simulink model "Refined_Model_42_VectoTnT"  (R2020b)
settings: Solver=FixedStepAuto  StartTime=0.0  StopTime=2500  FixedStep=dt  RelTol=1e-3
values from neighbouring files (symbols this model uses):
  ALInpSpeed = AxlLoss (1,:)    [GPS_val.m]    (also in ICEBEV_Script.m; ICEBEV_Script_VECTO.m; ICE_Script.m; ICE_Script_SSVal.m)
  ALInpTor = AxlLoss(:,1)    [GPS_val.m]    (also in ICEBEV_Script.m; ICEBEV_Script_VECTO.m; ICE_Script.m; ICE_Script_SSVal.m)
  ALTableVal = AxlLoss(2:end,2:end)    [GPS_val.m]    (also in ICEBEV_Script.m; ICEBEV_Script_VECTO.m; ICE_Script.m; ICE_Script_SSVal.m)
  CovDist = RoadProfile(:,4)    [ICE_Val.m]
  Cx = VehicleDefine(7,3)    [BEV_Basictest.m]    (also in GPS_val.m; ICEBEV_Script.m; ICEBEV_Script_VECTO.m; ICE_Script.m)
  Dist = 1:length(MaxSpeedProfile)    [GPS_val.m]    (also in ICE_Script.m; ICE_Val.m = [1:CovDist(end)])
  DynRolRad = VehicleDefine(5,3)    [BEV_Basictest.m]    (also in GPS_val.m; ICEBEV_Script.m; ICEBEV_Script_VECTO.m; ICE_Script.m)
  EngineRpm = round(IntpTorCur(:,1))    [GPS_val.m]    (also in ICEBEV_Script.m; ICEBEV_Script_VECTO.m; ICE_Script.m; ICE_Script_SSVal.m)
  EngineRpmRaw = TorCurRaw(:,1)    [GPS_val.m]    (also in ICEBEV_Script.m; ICEBEV_Script_VECTO.m; ICE_Script.m; ICE_Script_SSVal.m)
  etaClutch = VehicleDefine(23,3)    [GPS_val.m]    (also in ICEBEV_Script.m; ICEBEV_Script_VECTO.m; ICE_Script.m; ICE_Script_SSVal.m)
  FCTableVal = FCMap(2:end,2:end)    [GPS_val.m]    (also in ICEBEV_Script.m; ICEBEV_Script_VECTO.m; ICE_Script.m; ICE_Script_SSVal.m)
  FDR = VehicleDefine(20,3)    [BEV_Basictest.m]    (also in GPS_val.m = VehicleDefine(22,3); ICEBEV_Script.m = VehicleDefine(22,3); ICEBEV_Script_VECTO.m = VehicleDefine(22,3); ICE_Script.m = VehicleDefine(22,3))
  Fr = VehicleDefine(13,3)    [BEV_Basictest.m]    (also in GPS_val.m; ICEBEV_Script.m; ICEBEV_Script_VECTO.m; ICE_Script.m)
  g = VehicleDefine(14,3)    [BEV_Basictest.m]    (also in GPS_val.m; ICEBEV_Script.m; ICEBEV_Script_VECTO.m; ICE_Script.m)
  GNo = GBXDefine(:,1)    [GPS_val.m]    (also in ICEBEV_Script.m; ICEBEV_Script_VECTO.m; ICE_Script.m; ICE_Script_SSVal.m)
  GRa = GBXDefine(:,2)    [GPS_val.m]    (also in ICEBEV_Script.m; ICEBEV_Script_VECTO.m; ICE_Script.m; ICE_Script_SSVal.m)
  InitVel = VehicleDefine(21,3)    [BEV_Basictest.m]    (also in GPS_val.m = VehicleDefine(24,3); ICEBEV_Script.m = VehicleDefine(24,3); ICEBEV_Script_VECTO.m = VehicleDefine(24,3); ICE_Script.m = VehicleDefine(24,3))
  IntpSlope = round(IntpSlope,1)    [GPS_val.m]    (also in ICE_Script.m; ICE_Val.m = A)
  Je = VehicleDefine(25,3)    [GPS_val.m]    (also in ICEBEV_Script.m; ICEBEV_Script_VECTO.m; ICE_Script.m; ICE_Script_SSVal.m)
  Jk = VehicleDefine(15,3)    [BEV_Basictest.m]    (also in GPS_val.m; ICEBEV_Script.m; ICEBEV_Script_VECTO.m; ICE_Script.m)
  Jm = VehicleDefine(16,3)    [GPS_val.m]    (also in ICEBEV_Script.m; ICEBEV_Script_VECTO.m; ICE_Script.m; ICE_Script_SSVal.m)
  MaxAcc = 1    [BEV_Basictest.m]    (also in GPS_val.m; ICEBEV_Script.m; ICEBEV_Script_VECTO.m; ICE_Script.m)
  MaxDec = 1    [BEV_Basictest.m]    (also in GPS_val.m; ICEBEV_Script.m; ICEBEV_Script_VECTO.m; ICE_Script.m)
  MaxSpeedProfile = FMSP    [GPS_val.m]    (also in ICE_Script.m; ICE_Val.m = repelem(SegSPLatinmps,SegLeninm))
  MaxTorValThrot = max(ThrotTableVal,[],2)    [GPS_val.m]    (also in ICEBEV_Script.m; ICEBEV_Script_VECTO.m; ICE_Script.m; ICE_Script_SSVal.m)
  Me = VehicleDefine(10,3)    [BEV_Basictest.m]    (also in GPS_val.m; ICEBEV_Script.m; ICEBEV_Script_VECTO.m; ICE_Script.m)
  MotoringTor = IntpTorCur(:,3)    [GPS_val.m]    (also in ICEBEV_Script.m; ICEBEV_Script_VECTO.m; ICE_Script.m; ICE_Script_SSVal.m)
  Mt = VehicleDefine(12,3)    [BEV_Basictest.m]    (also in GPS_val.m; ICEBEV_Script.m; ICEBEV_Script_VECTO.m; ICE_Script.m)
  Mtot = Mv+Me+Mt    [BEV_Basictest.m]    (also in GPS_val.m; ICEBEV_Script.m; ICEBEV_Script_VECTO.m; ICE_Script.m)
  Mv = VehicleDefine(9,3)    [BEV_Basictest.m]    (also in GPS_val.m; ICEBEV_Script.m; ICEBEV_Script_VECTO.m; ICE_Script.m)
  NoSteps = round(Dist(end))    [GPS_val.m]    (also in ICE_Script.m; ICE_Val.m = 3002)
  NoWhlFA = VehicleDefine(2,3)    [BEV_Basictest.m]    (also in GPS_val.m; ICE_Script.m; ICE_Val.m; ICE_Val_new.m)
  NoWhlRA = VehicleDefine(4,3)    [BEV_Basictest.m]    (also in GPS_val.m; ICE_Script.m; ICE_Val.m; ICE_Val_new.m)
  rho = VehicleDefine(6,3)    [BEV_Basictest.m]    (also in GPS_val.m; ICEBEV_Script.m; ICEBEV_Script_VECTO.m; ICE_Script.m)
  RpmBrkPnt = ThrottleMap(1,:)    [GPS_val.m]    (also in ICEBEV_Script.m; ICEBEV_Script_VECTO.m; ICE_Script.m; ICE_Script_SSVal.m)
  s = divisors(length(MaxSpeedProfile))    [GPS_val.m]    (also in ICEBEV_Script.m = round(FLoadTor); ICEBEV_Script_VECTO.m = round(FLoadTor); ICE_Script.m = round(FLoadTor); ICE_Script_SSVal.m = round(FLoadTor))
  SegNo = RoadProfile(:,1)    [ICE_Val.m]
  SegSPLatinmps = (sqrt(aMaxLat*g*CurRadinm))    [GPS_val.m]    (also in ICE_Script.m; ICE_Val.m)
  Sx = VehicleDefine(8,3)    [BEV_Basictest.m]    (also in GPS_val.m; ICEBEV_Script.m; ICEBEV_Script_VECTO.m; ICE_Script.m)
  ThrotPos = ThrotPos'    [GPS_val.m]    (also in ICEBEV_Script.m; ICEBEV_Script_VECTO.m; ICE_Script.m; ICE_Script_SSVal.m)
  ThrotTableVal = ThrottleMap(2:end,2:end)    [GPS_val.m]    (also in ICEBEV_Script.m; ICEBEV_Script_VECTO.m; ICE_Script.m; ICE_Script_SSVal.m)
undefined symbols (not defined in the file or in its folder): G1Inprpm, GearNo, GInprpm, GInpTor, GTorLoss, MaxSpinG, MaxWhlTorinG, Stoptimes
libraries: simulink x4, autolibshared x1
settings Model: Creator=Kshitij  LastModifiedBy=Kshitij
settings DebuggingCC: AlgebraicLoopMsg=none

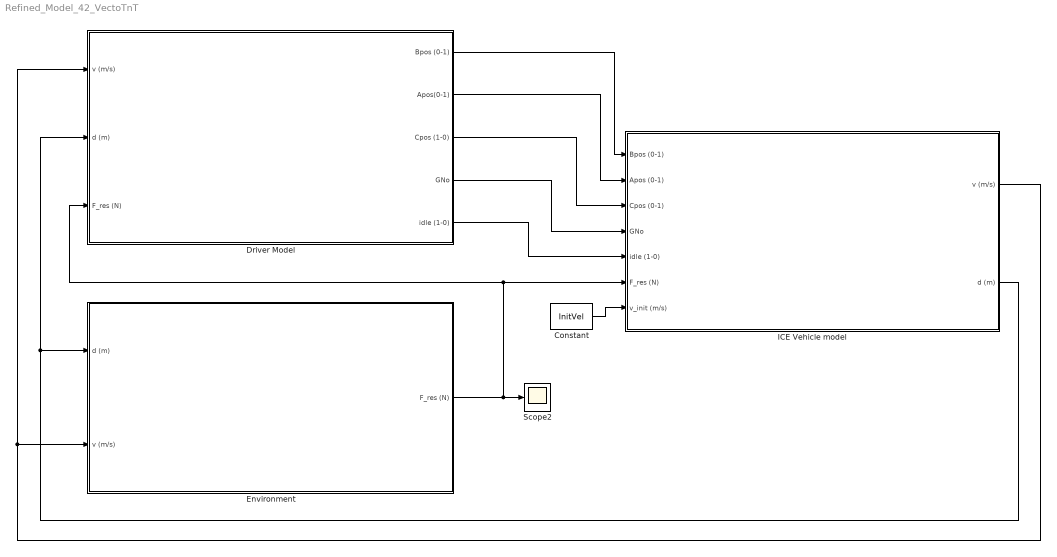
== system Refined_Model_42_VectoTnT ==
  Constant : Constant  Value=InitVel
  Driver Model : Subsystem
  Environment : Subsystem
  ICE Vehicle model : Subsystem
  Scope2 : Scope
  wires:
  Environment/1(F_res (N)) -> Driver Model/3(F_res (N)), ICE Vehicle model/6(F_res (N)), Scope2/1
  Constant/1 -> ICE Vehicle model/7(v_init (m/s))
  Driver Model/3(Cpos (1-0)) -> ICE Vehicle model/3(Cpos (0-1))
  Driver Model/4(GNo) -> ICE Vehicle model/4(GNo)
  Driver Model/2(Apos(0-1)) -> ICE Vehicle model/2(Apos (0-1))
  ICE Vehicle model/1(v (m/s)) -> Environment/2(v (m/s)), Driver Model/1(v (m/s))
  ICE Vehicle model/2(d (m)) -> Environment/1(d (m)), Driver Model/2(d (m))
  Driver Model/5(idle (1-0)) -> ICE Vehicle model/5(idle (1-0))
  Driver Model/1(Bpos (0-1)) -> ICE Vehicle model/1(Bpos (0-1))

== system Refined_Model_42_VectoTnT/Driver Model ==
  v (m/s) : Inport
  d (m) : Inport  Port=2
  F_res (N) : Inport  Port=3
  Acc/Dec Control : Subsystem
  Driver Throttle Mapping ICE : Subsystem
  Gear and Clutch Definition : Subsystem
  Bpos (0-1) : Outport
  Apos(0-1) : Outport  Port=2
  Cpos (1-0) : Outport  Port=3
  GNo : Outport  Port=4
  idle (1-0) : Outport  Port=5
  wires:
  Acc/Dec Control/2(Bpos (0-1)) -> Bpos (0-1)/1
  d (m)/1 -> Acc/Dec Control/2(d (m))
  Gear and Clutch Definition/1(Cpos) -> Cpos (1-0)/1
  Gear and Clutch Definition/2(GNo) -> Driver Throttle Mapping ICE/1(GNo), GNo/1
  Driver Throttle Mapping ICE/1(T_w_req (Nm)) -> Gear and Clutch Definition/1(T_w_req (Nm))  "T_w_req (Nm)"
  F_res (N)/1 -> Driver Throttle Mapping ICE/2(F_res (N))  "F_res (N)"
  Acc/Dec Control/3(Arate(0-1)) -> Driver Throttle Mapping ICE/3(Arate(0-1))
  Driver Throttle Mapping ICE/2(Apos (0-1)) -> Apos(0-1)/1
  v (m/s)/1 -> Acc/Dec Control/1(v (m/s)), Gear and Clutch Definition/2(v (m/s))
  Acc/Dec Control/1(idle (0-1)) -> Gear and Clutch Definition/3(idle (0-1)), idle (1-0)/1

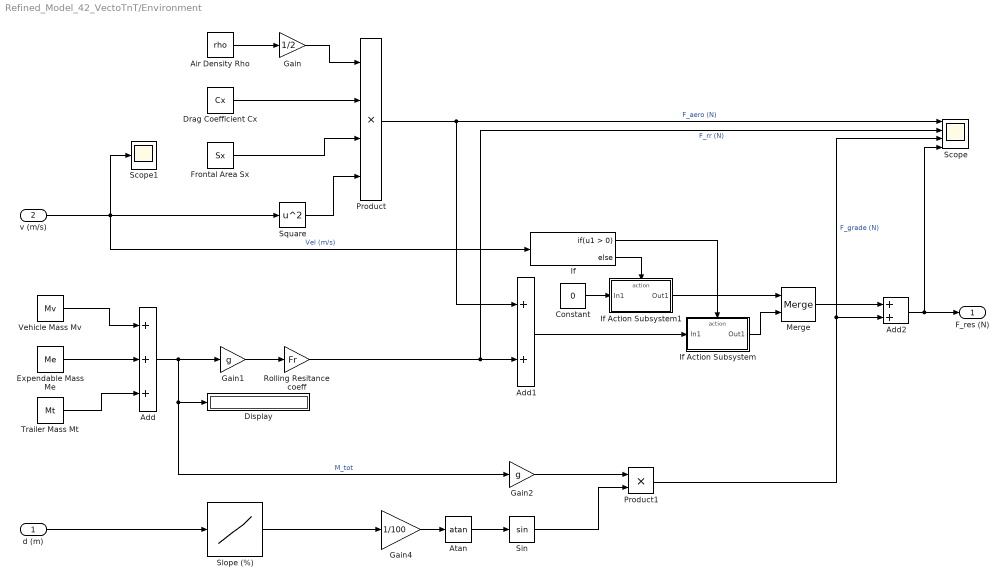
== system Refined_Model_42_VectoTnT/Environment ==
  d (m) : Inport
  v (m/s) : Inport  Port=2
  Add : Sum  Inputs=+++
  Add1 : Sum
  Add2 : Sum
  Air Density Rho : Constant  Value=rho
  Atan : Trigonometry  Operator=atan
  Constant : Constant  Value=0
  Display : Display
  Drag Coefficient Cx : Constant  Value=Cx
  Expendable Mass Me : Constant  Value=Me
  Frontal Area Sx : Constant  Value=Sx
  Gain : Gain  Gain=1/2
  Gain1 : Gain  Gain=g
  Gain2 : Gain  Gain=g
  Gain4 : Gain  Gain=1/100
  If : If
  If Action Subsystem : Subsystem  TreatAsAtomicUnit=on
  If Action Subsystem1 : Subsystem  TreatAsAtomicUnit=on
  Merge : Merge
  Product : Product  Inputs=4
  Product1 : Product
  Rolling Resitance coeff : Gain  Gain=Fr
  Scope : Scope  NumInputPorts=4
  Scope1 : Scope
  Sin : Trigonometry
  Slope (%) : Lookup_n-D  NumberOfTableDimensions=1  BreakpointsForDimension1=Dist  Table=IntpSlope  InternalRulePriority=Speed  RndMeth=Simplest  InputSameDT=on
  Square : Math  Operator=square  SaturateOnIntegerOverflow=on
  Trailer Mass Mt : Constant  Value=Mt
  Vehicle Mass Mv : Constant  Value=Mv
  F_res (N) : Outport
  wires:
  Expendable Mass Me/1 -> Add/2
  Add/1 -> Gain2/1, Display/1, Gain1/1  "M_tot"
  Gain/1 -> Product/1
  Sin/1 -> Product1/2
  Product1/1 -> Scope/3, Add2/2  "F_grade (N)"
  Air Density Rho/1 -> Gain/1
  Drag Coefficient Cx/1 -> Product/2
  v (m/s)/1 -> Scope1/1, Square/1, If/1  "Vel (m/s)"
  d (m)/1 -> Slope (%)/1
  Gain2/1 -> Product1/1
  Trailer Mass Mt/1 -> Add/3
  Rolling Resitance coeff/1 -> Scope/2, Add1/2  "F_rr (N)"
  Square/1 -> Product/4
  Gain1/1 -> Rolling Resitance coeff/1
  Vehicle Mass Mv/1 -> Add/1
  Product/1 -> Scope/1, Add1/1  "F_aero (N)"
  Frontal Area Sx/1 -> Product/3
  If/1 -> If Action Subsystem/Action
  If/2 -> If Action Subsystem1/Action
  If Action Subsystem1/1(Out1) -> Merge/1
  Add1/1 -> If Action Subsystem/1(In1)
  If Action Subsystem/1(Out1) -> Merge/2
  Constant/1 -> If Action Subsystem1/1(In1)
  Merge/1 -> Add2/1
  Add2/1 -> F_res (N)/1, Scope/4
  Slope (%)/1 -> Gain4/1
  Atan/1 -> Sin/1
  Gain4/1 -> Atan/1

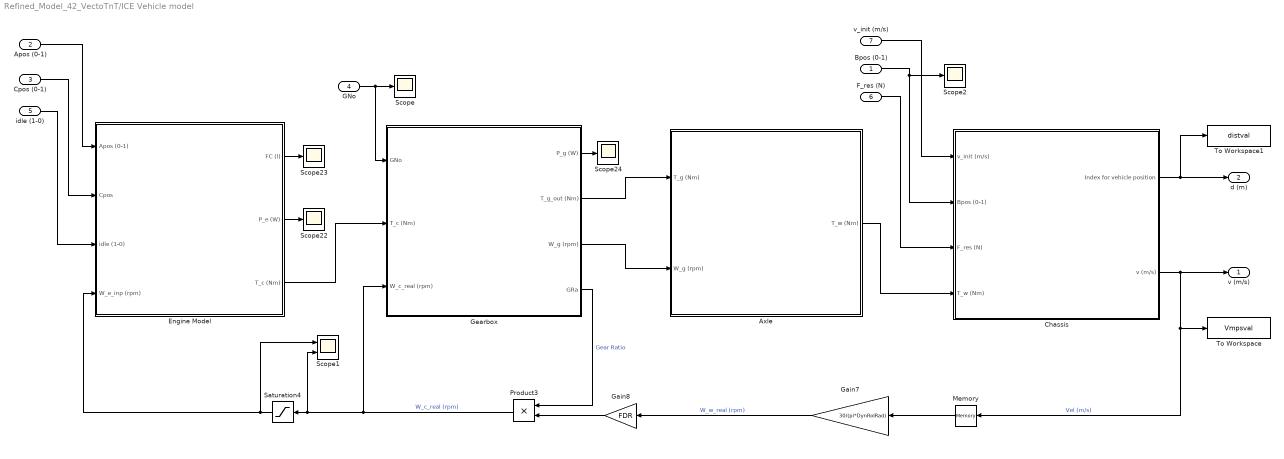
== system Refined_Model_42_VectoTnT/ICE Vehicle model ==
  Bpos (0-1) : Inport
  Apos (0-1) : Inport  Port=2
  Cpos (0-1) : Inport  Port=3
  GNo : Inport  Port=4
  idle (1-0) : Inport  Port=5
  F_res (N) : Inport  Port=6
  v_init (m/s) : Inport  Port=7
  Axle : Subsystem
  Chassis : Subsystem
  Engine Model : Subsystem
  Gain7 : Gain  Gain=30/(pi*DynRolRad)
  Gain8 : Gain  Gain=FDR
  Gearbox : Subsystem
  Memory : Memory
  Product3 : Product
  Saturation4 : Saturate  UpperLimit=max(EngineRpmRaw)  LowerLimit=min(EngineRpmRaw)
  Scope{,2,22..24} (5 alike) : Scope
  Scope1 : Scope  NumInputPorts=2
  To Workspace : ToWorkspace  VariableName=Vmpsval  SaveFormat=Timeseries  SampleTime=-1
  To Workspace1 : ToWorkspace  VariableName=distval  SaveFormat=Timeseries  SampleTime=-1
  v (m/s) : Outport
  d (m) : Outport  Port=2
  wires:
  Gearbox/2(T_g_out (Nm)) -> Axle/1(T_g (Nm))
  Chassis/1(Index for vehicle position) -> To Workspace1/1, d (m)/1
  Bpos (0-1)/1 -> Chassis/2(Bpos (0-1)), Scope2/1
  v_init (m/s)/1 -> Chassis/1(v_init (m/s))
  Axle/1(T_w (Nm)) -> Chassis/4(T_w (Nm))
  F_res (N)/1 -> Chassis/3(F_res (N))
  Gearbox/1(P_g (W)) -> Scope24/1
  Engine Model/3(T_c (Nm)) -> Gearbox/2(T_c (Nm))
  Apos (0-1)/1 -> Engine Model/1(Apos (0-1))
  Engine Model/2(P_e (W)) -> Scope22/1
  Engine Model/1(FC (l)) -> Scope23/1
  GNo/1 -> Gearbox/1(GNo), Scope/1
  Chassis/2(v (m/s)) -> v (m/s)/1, Memory/1, To Workspace/1  "Vel (m/s)"
  Gearbox/4(GRa) -> Product3/1  "Gear Ratio"
  Gain8/1 -> Product3/2
  Gain7/1 -> Gain8/1  "W_w_real (rpm)"
  Cpos (0-1)/1 -> Engine Model/2(Cpos)
  Product3/1 -> Scope1/2, Saturation4/1, Gearbox/3(W_c_real (rpm))  "W_c_real (rpm)"
  Saturation4/1 -> Scope1/1, Engine Model/4(W_e_inp (rpm))
  Memory/1 -> Gain7/1
  idle (1-0)/1 -> Engine Model/3(idle (1-0))
  Gearbox/3(W_g (rpm)) -> Axle/2(W_g (rpm))

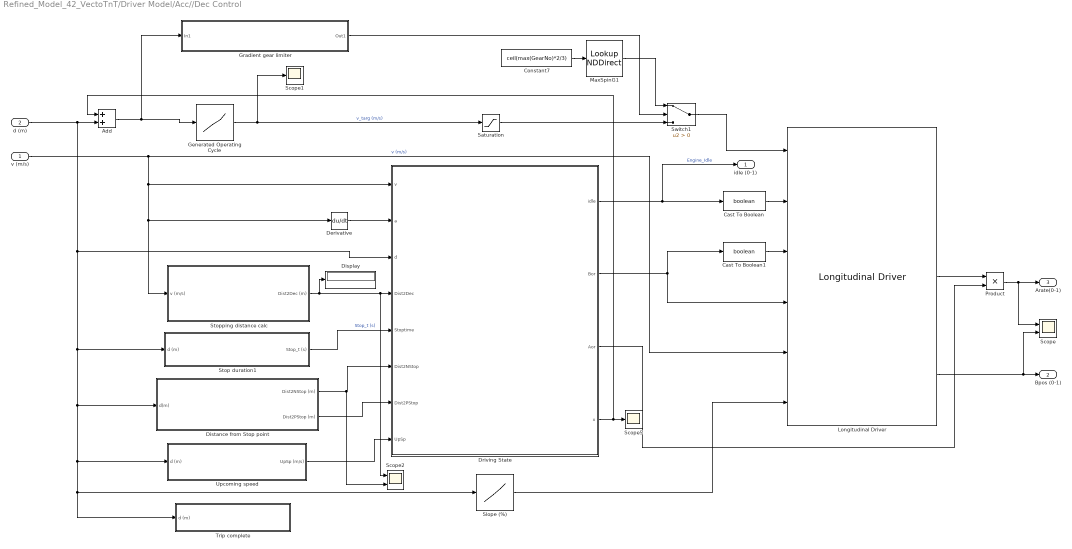
== system Refined_Model_42_VectoTnT/Driver Model/Acc//Dec Control ==
  v (m/s) : Inport
  d (m) : Inport  Port=2
  Add : Sum
  Cast To Boolean : DataTypeConversion  OutDataTypeStr=boolean
  Cast To Boolean1 : DataTypeConversion  OutDataTypeStr=boolean
  Constant7 : Constant  Value=ceil(max(GearNo)*2/3)
  Derivative : Derivative
  Display : Display
  Distance from Stop point : Subsystem
  Driving State : Stateflow chart  TreatAsAtomicUnit=on
      settings: PortSchema="{\"entries\":[{\"content\":{\"sides\":[{\"content\":{\"connectorIds\":[\"In1\",\"In2\",\"In3\",\"In6\",\"In4\",\"In5\",\"In8\",\"In7\"]},\"type\":\"ConnectorPlacement.EquallySpacedRectSide\",\"uuid\":\"d08c6342-d75c-4cbe-aad4-154711b37fb2\"},{\"content\":{\"connectorIds\":[\"Out1\",\"Out2\",\"Out3\",\"Out4\"],\"side\":\"RIGHT\"},\"type\":\"ConnectorPlacement.EquallySpacedRectSide\",\"uuid\":\"8a1951a0-5a37-479b-8286-6923b1e8a7ed\"},{\"content\":{\"connectorIds\":[],\"side\":\"TOP\"},\"type\":\"ConnectorPlacement.EquallySpacedRectSide\",\"uuid\":\"4f69c596-a605-4847-b163-f2b0badabc3a\"},{\"content\":{\"connectorIds\":[],\"side\":\"HIDDEN\"},\"type\":\"ConnectorPlacement.EquallySpacedRectSide\",\"uuid\":\"cbb16f2b-3903-4d38-b3c0-6da7c4a6c3c0\"}]},\"type\":\"ConnectorPlacement.EquallySpacedConnector\",\"uuid\":\"76dd4822-1d6a-4887-906b-ffb42e8ecb43\"}],\"packageUris\":[\"http://schema.mathworks.com/mf0/Connector/R2020b\"],\"version\":\"1.0\"}"
  Generated Operating Cycle : Lookup_n-D  NumberOfTableDimensions=1  BreakpointsForDimension1=Dist  BreakpointsForDimension2=G1Inprpm  Table=MaxSpeedProfile  InterpMethod=Linear Lagrange  InternalRulePriority=Speed  RndMeth=Simplest  InputSameDT=on
  Gradient gear limiter : Subsystem
  Longitudinal Driver : autolibshared/Longitudinal Driver  extAccelOvr=off  extDecelOvr=on  extAccelHld=off  extDecelHld=off  extAccelZero=on  extDecelZero=off  cntrlType=PI  shftType=None  velUnits=m/s  gearOut=off  Kp=200  Ki=175  Kff=0  Kg=0  VehVelVec=[0 100]  KffVec=[.1 .1]  KpVec=[10 10]  KiVec=[5 5]  KgVec=[0 0]  m=1500  Kpt=3000  tau=.1  L=2  aR=200  bR=2.5  cR=.5  g=9.81  vnom=100  Kaw=0  tauerr=0  tauPt=2  GearInit=0  tShift=.1  pdlVec=[0.1 0.4 0.5 0.9]  upShftTbl=[-1 12.9375 26.4375 39.9375 51.18749999999999 62.4375 72.84375 83.25;-1 16.3125 29.8125 43.3125 54.5624 65.8125 76.78125 87.75;-1 19.6875 33.1875 46.68749999999999 57.9375 69.1875 80.71875 92.25;-1 33 52.5 77.25 100.5 138.75 161.875 185]  dwnShftTbl=[1 9.5625 23.0625 36.5625 47.8125 59.0625 68.90625 78.75;1 12.9375 26.4375 39.9375 51.18749999999999 62.4375 72.84375 83.25;1 16.3125 29.8125 43.3125 54.562499 65.8125 76.78125 87.75;1 19.6875 33.1875 46.68749999999999 57.9375 69.1875 80.71875 92.25]  tClutch=.5  tRev=.5  tPark=120  aMode=1  UpGearVec="[0  1  2  3  4  5  6  7]"  DownGearVec="[1  2  3  4  5  6  7  8]"
      settings: SourceProductBaseCode=PW,MT,UV,VE,VP
  MaxSpinG1 : LookupNDDirect  NumberOfTableDimensions=1  Table=MaxSpinG
  Product : Product
  Saturation : Saturate  UpperLimit=inf  LowerLimit=0
  Scope : Scope  NumInputPorts=2
  Scope1 : Scope
  Scope2 : Scope  NumInputPorts=2
  Scope5 : Scope
  Slope (%) : Lookup_n-D  NumberOfTableDimensions=1  BreakpointsForDimension1=Dist  Table=IntpSlope  InternalRulePriority=Speed  RndMeth=Simplest  InputSameDT=on
  Stop duration1 : Subsystem
  Stopping distance calc : Subsystem
  Switch1 : Switch  Criteria=u2 > Threshold
  Trip complete : Subsystem
  Upcoming speed : Subsystem
  idle (0-1) : Outport
  Bpos (0-1) : Outport  Port=2
  Arate(0-1) : Outport  Port=3
  wires:
  Cast To Boolean1/1 -> Longitudinal Driver/3
  Driving State/1(idle) -> Cast To Boolean/1, idle (0-1)/1  "Engine_Idle"
  Derivative/1 -> Driving State/2(a)
  Upcoming speed/1(UpSp (m/s)) -> Driving State/7(UpSp)
  Stopping distance calc/1(Dist2Dec (m)) -> Display/1, Scope2/1, Driving State/6(Dist2Dec)
  Stop duration1/1(Stop_t (s)) -> Driving State/4(Stoptime)  "Stop_t (s)"
  Driving State/2(Bor) -> Cast To Boolean1/1, Longitudinal Driver/4
  Slope (%)/1 -> Longitudinal Driver/6
  Cast To Boolean/1 -> Longitudinal Driver/2
  Longitudinal Driver/2 -> Product/1
  Longitudinal Driver/3 -> Scope/2, Bpos (0-1)/1
  Generated Operating Cycle/1 -> Saturation/1, Scope1/1  "v_targ (m/s)"
  v (m/s)/1 -> Driving State/1(v), Stopping distance calc/1(v (m/s)), Derivative/1, Longitudinal Driver/5  "v (m/s)"
  d (m)/1 -> Add/2, Stop duration1/1(d (m)), Trip complete/1(d (m)), Slope (%)/1, Upcoming speed/1(d (m)), Distance from Stop point/1(d(m)), Driving State/3(d)
  Driving State/3(Aor) -> Product/2
  Product/1 -> Scope/1, Arate(0-1)/1
  Distance from Stop point/1(Dist2NStop (m)) -> Scope2/2, Driving State/5(Dist2NStop)
  Distance from Stop point/2(Dist2PStop (m)) -> Driving State/8(Dist2PStop)
  Driving State/4(x) -> Add/1, Scope5/1
  Add/1 -> Gradient gear limiter/1(In1), Generated Operating Cycle/1
  Constant7/1 -> MaxSpinG1/1
  Saturation/1 -> Switch1/3
  Switch1/1 -> Longitudinal Driver/1
  MaxSpinG1/1 -> Switch1/1
  Gradient gear limiter/1(Out1) -> Switch1/2

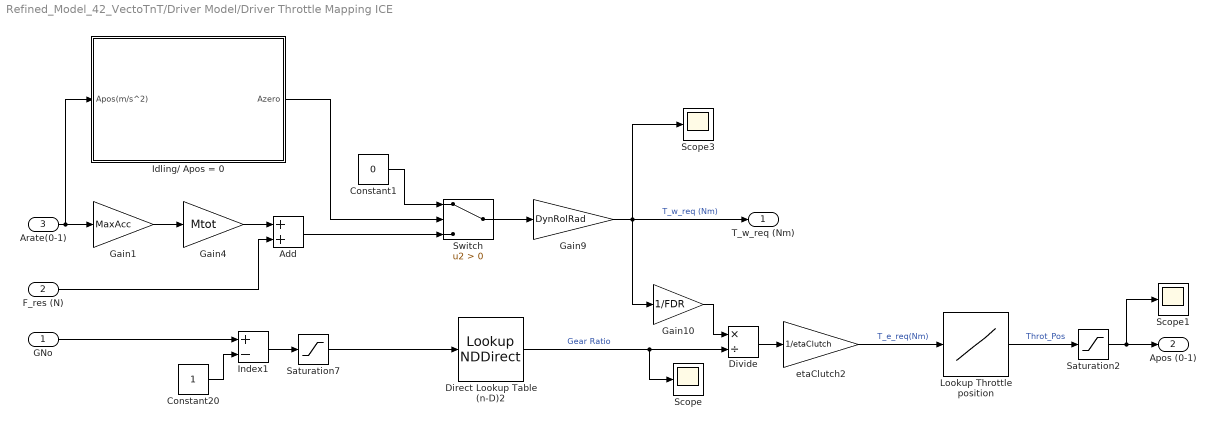
== system Refined_Model_42_VectoTnT/Driver Model/Driver Throttle Mapping ICE ==
  GNo : Inport
  F_res (N) : Inport  Port=2
  Arate(0-1) : Inport  Port=3
  Add : Sum
  Constant1 : Constant  Value=0
  Constant20 : Constant
  Direct Lookup Table (n-D)2 : LookupNDDirect  NumberOfTableDimensions=1  Table=GRa
  Divide : Product  Inputs=*/
  Gain1 : Gain  Gain=MaxAcc
  Gain10 : Gain  Gain=1/FDR
  Gain4 : Gain  Gain=Mtot
  Gain9 : Gain  Gain=DynRolRad
  Idling/ Apos = 0 : Subsystem
  Index1 : Sum  Inputs=+-
  Lookup Throttle position : Lookup_n-D  NumberOfTableDimensions=1  BreakpointsForDimension1=MaxTorValThrot  Table=ThrotPos  InternalRulePriority=Speed  RndMeth=Simplest  InputSameDT=on
  Saturation2 : Saturate  UpperLimit=1  LowerLimit=0
  Saturation7 : Saturate  UpperLimit=inf  LowerLimit=0
  Scope : Scope
  Scope1 : Scope
  Scope3 : Scope
  Switch : Switch  Criteria=u2 > Threshold
  etaClutch2 : Gain  Gain=1/etaClutch
  T_w_req (Nm) : Outport
  Apos (0-1) : Outport  Port=2
  wires:
  etaClutch2/1 -> Lookup Throttle position/1  "T_e_req(Nm)"
  Add/1 -> Switch/3
  Gain9/1 -> Scope3/1, T_w_req (Nm)/1, Gain10/1  "T_w_req (Nm)"
  Gain10/1 -> Divide/1
  Gain4/1 -> Add/1
  Divide/1 -> etaClutch2/1
  F_res (N)/1 -> Add/2
  Lookup Throttle position/1 -> Saturation2/1  "Throt_Pos"
  Saturation2/1 -> Apos (0-1)/1, Scope1/1
  Arate(0-1)/1 -> Idling/ Apos = 0/1(Apos(m/s^2)), Gain1/1
  Gain1/1 -> Gain4/1
  Constant20/1 -> Index1/2
  GNo/1 -> Index1/1
  Index1/1 -> Saturation7/1
  Saturation7/1 -> Direct Lookup Table (n-D)2/1
  Direct Lookup Table (n-D)2/1 -> Scope/1, Divide/2  "Gear Ratio"
  Switch/1 -> Gain9/1
  Constant1/1 -> Switch/1
  Idling/ Apos = 0/1(Azero) -> Switch/2

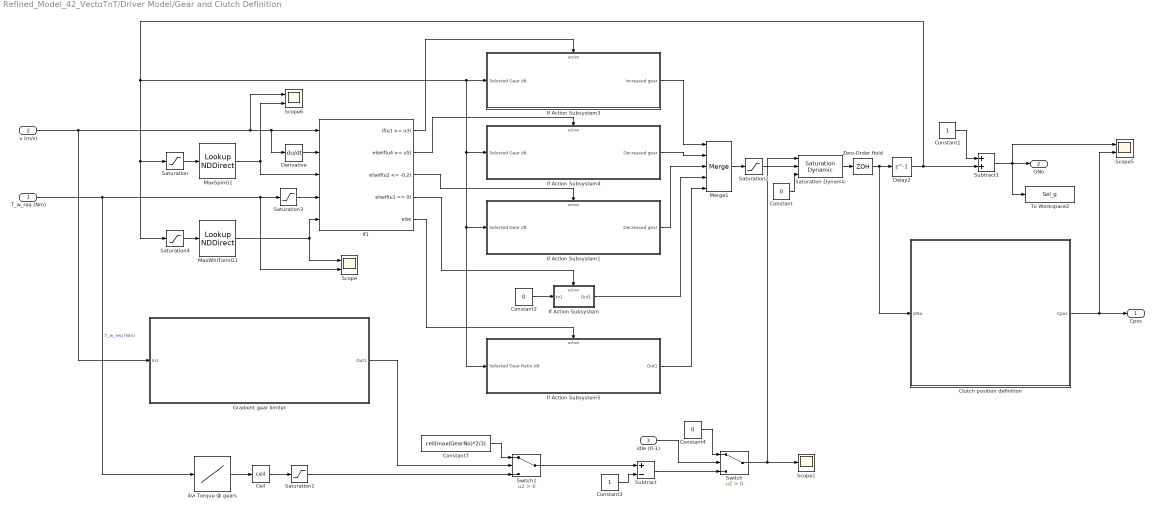
== system Refined_Model_42_VectoTnT/Driver Model/Gear and Clutch Definition ==
  T_w_req (Nm) : Inport
  v (m/s) : Inport  Port=2
  idle (0-1) : Inport  Port=3
  Avl Torque @ gears : Lookup_n-D  NumberOfTableDimensions=1  BreakpointsForDimension1=flip(MaxWhlTorinG)  Table=flip(GNo)  InternalRulePriority=Speed  RndMeth=Simplest  InputSameDT=on
  Ceil : Rounding  Operator=ceil
  Clutch position definition : Subsystem
  Constant : Constant  Value=0
  Constant1 : Constant
  Constant2 : Constant  Value=0
  Constant3 : Constant
  Constant4 : Constant  Value=0
  Constant7 : Constant  Value=ceil(max(GearNo)*2/3)
  Delay2 : Delay  DelayLength=1
  Derivative : Derivative
  Gradient gear limiter : Subsystem
  If Action Subsystem : Subsystem  TreatAsAtomicUnit=on
  If Action Subsystem1 : Subsystem  TreatAsAtomicUnit=on
  If Action Subsystem3 : Subsystem  TreatAsAtomicUnit=on
  If Action Subsystem4 : Subsystem  TreatAsAtomicUnit=on
  If Action Subsystem5 : Subsystem  TreatAsAtomicUnit=on
  If1 : If  NumInputs=5  IfExpression=u1 >= u3  ElseIfExpressions=u4 >= u5 ,u2 <= -0.2, u1 == 0
  MaxSpinG1 : LookupNDDirect  NumberOfTableDimensions=1  Table=MaxSpinG
  MaxWhlTorinG1 : LookupNDDirect  NumberOfTableDimensions=1  Table=MaxWhlTorinG
  Merge1 : Merge  Inputs=5
  Saturation : Saturate  UpperLimit=inf  LowerLimit=0
  Saturation Dynamic : simulink/Discontinuities/Saturation Dynamic  OutMin=[]  OutMax=[]  OutDataTypeStr=Inherit: Same as second input  OutDataType=fixdt(1, 16)  OutScaling=2^-10  DoSatur=off
  Saturation1 : Saturate  UpperLimit=max(GNo)  LowerLimit=0
  Saturation2 : Saturate  UpperLimit=max(GNo)-1  LowerLimit=0
  Saturation3 : Saturate  UpperLimit=inf  LowerLimit=0
  Saturation4 : Saturate  UpperLimit=inf  LowerLimit=0
  Scope : Scope  NumInputPorts=2
  Scope1 : Scope
  Scope5 : Scope  NumInputPorts=2
  Scope6 : Scope  NumInputPorts=2
  Subtract : Sum  Inputs=+-
  Subtract1 : Sum
  Switch : Switch  Criteria=u2 > Threshold
  Switch1 : Switch  Criteria=u2 > Threshold
  To Workspace2 : ToWorkspace  VariableName=Sel_g  SaveFormat=Timeseries  SampleTime=-1
  Zero-Order Hold : ZeroOrderHold  SampleTime=15
  Cpos : Outport
  GNo : Outport  Port=2
  wires:
  Clutch position definition/1(Cpos) -> Scope5/2, Cpos/1
  If1/2 -> If Action Subsystem4/Action
  If Action Subsystem4/1(Decreased gear) -> Merge1/2
  If1/5 -> If Action Subsystem5/Action
  If Action Subsystem3/1(Increased gear) -> Merge1/1
  MaxSpinG1/1 -> If1/3, Scope6/2
  If Action Subsystem5/1(Out1) -> Merge1/5
  MaxWhlTorinG1/1 -> If1/5, Scope/1
  If1/1 -> If Action Subsystem3/Action
  Saturation3/1 -> If1/4
  T_w_req (Nm)/1 -> Avl Torque @ gears/1, Scope/2, Saturation3/1  "T_w_req (Nm)"
  Constant1/1 -> Subtract1/1
  Saturation/1 -> MaxSpinG1/1
  Saturation4/1 -> MaxWhlTorinG1/1
  Delay2/1 -> Subtract1/2, If Action Subsystem3/1(Selected Gear /dt), If Action Subsystem1/1(Selected Gear /dt), If Action Subsystem5/1(Selected Gear Ratio /dt), If Action Subsystem4/1(Selected Gear /dt), Saturation/1, Saturation4/1
  Subtract1/1 -> Scope5/1, GNo/1, To Workspace2/1
  v (m/s)/1 -> Gradient gear limiter/1(In1), Derivative/1, If1/1, Scope6/1
  If1/3 -> If Action Subsystem1/Action
  If Action Subsystem1/1(Decreased gear) -> Merge1/3
  Merge1/1 -> Saturation2/1
  Avl Torque @ gears/1 -> Ceil/1
  Ceil/1 -> Saturation1/1
  Saturation Dynamic/1 -> Zero-Order Hold/1
  Constant3/1 -> Subtract/2
  Switch1/1 -> Subtract/1
  Saturation2/1 -> Saturation Dynamic/2
  Constant/1 -> Saturation Dynamic/3
  Switch/1 -> Saturation Dynamic/1, Scope1/1
  Zero-Order Hold/1 -> Delay2/1, Clutch position definition/1(GNo)
  Derivative/1 -> If1/2
  If1/4 -> If Action Subsystem/Action
  Constant2/1 -> If Action Subsystem/1(In1)
  If Action Subsystem/1(Out1) -> Merge1/4
  Subtract/1 -> Switch/3
  idle (0-1)/1 -> Switch/2
  Constant4/1 -> Switch/1
  Saturation1/1 -> Switch1/3
  Constant7/1 -> Switch1/1
  Gradient gear limiter/1(Out1) -> Switch1/2

== system Refined_Model_42_VectoTnT/Environment/If Action Subsystem ==
  In1 : Inport
  Action Port : ActionPort  ActionPortLabel=if(u1 > 0)
  Out1 : Outport
  wires:
  In1/1 -> Out1/1

== system Refined_Model_42_VectoTnT/Environment/If Action Subsystem1 ==
  In1 : Inport
  Action Port : ActionPort  ActionPortLabel=else
  Out1 : Outport
  wires:
  In1/1 -> Out1/1

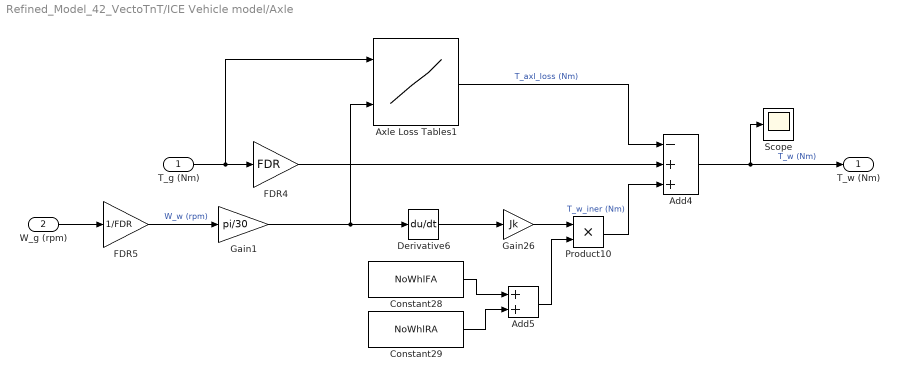
== system Refined_Model_42_VectoTnT/ICE Vehicle model/Axle ==
  T_g (Nm) : Inport
  W_g (rpm) : Inport  Port=2
  Add4 : Sum  Inputs=-++
  Add5 : Sum
  Axle Loss Tables1 : Lookup_n-D  BreakpointsForDimension1=ALInpTor  BreakpointsForDimension2=ALInpSpeed  BreakpointsForDimension3=GNo  Table=ALTableVal  InterpMethod=Linear Lagrange  InternalRulePriority=Speed  RndMeth=Simplest  InputSameDT=on
      settings: InputPortMap=u0,u1
  Constant28 : Constant  Value=NoWhlFA
  Constant29 : Constant  Value=NoWhlRA
  Derivative6 : Derivative
  FDR4 : Gain  Gain=FDR
  FDR5 : Gain  Gain=1/FDR
  Gain1 : Gain  Gain=pi/30
  Gain26 : Gain  Gain=Jk
  Product10 : Product
  Scope : Scope
  T_w (Nm) : Outport
  wires:
  Product10/1 -> Add4/3  "T_w_iner (Nm)"
  Derivative6/1 -> Gain26/1
  Add5/1 -> Product10/2
  Constant29/1 -> Add5/2
  Constant28/1 -> Add5/1
  FDR4/1 -> Add4/2
  Gain26/1 -> Product10/1
  Add4/1 -> T_w (Nm)/1, Scope/1  "T_w (Nm)"
  T_g (Nm)/1 -> Axle Loss Tables1/1, FDR4/1
  Axle Loss Tables1/1 -> Add4/1  "T_axl_loss (Nm)"
  Gain1/1 -> Axle Loss Tables1/2, Derivative6/1
  W_g (rpm)/1 -> FDR5/1
  FDR5/1 -> Gain1/1  "W_w (rpm)"

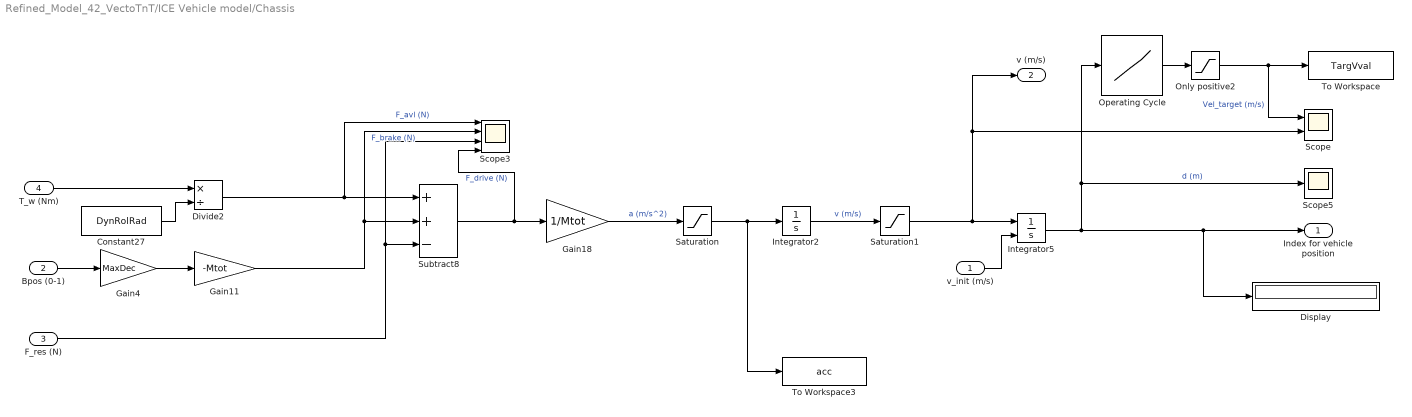
== system Refined_Model_42_VectoTnT/ICE Vehicle model/Chassis ==
  v_init (m/s) : Inport
  Bpos (0-1) : Inport  Port=2
  F_res (N) : Inport  Port=3
  T_w (Nm) : Inport  Port=4
  Constant27 : Constant  Value=DynRolRad
  Display : Display
  Divide2 : Product  Inputs=*/
  Gain11 : Gain  Gain=-Mtot
  Gain18 : Gain  Gain=1/Mtot
  Gain4 : Gain  Gain=MaxDec
  Integrator2 : Integrator  ContinuousStateAttributes='acceleration'
  Integrator5 : Integrator  InitialConditionSource=external  ContinuousStateAttributes='velocity'
  Only positive2 : Saturate  UpperLimit=inf  LowerLimit=0
  Operating Cycle : Lookup_n-D  NumberOfTableDimensions=1  BreakpointsForDimension1=Dist  BreakpointsForDimension2=G1Inprpm  Table=MaxSpeedProfile  InterpMethod=Linear Lagrange  InternalRulePriority=Speed  RndMeth=Simplest  InputSameDT=on
  Saturation : Saturate  UpperLimit=MaxAcc  LowerLimit=-(MaxDec)
  Saturation1 : Saturate  UpperLimit=inf  LowerLimit=0
  Scope : Scope  NumInputPorts=2
  Scope3 : Scope  NumInputPorts=4
  Scope5 : Scope
  Subtract8 : Sum  Inputs=++-
  To Workspace : ToWorkspace  VariableName=TargVval  SaveFormat=Timeseries  SampleTime=-1
  To Workspace3 : ToWorkspace  VariableName=acc  SaveFormat=Timeseries  SampleTime=-1
  Index for vehicle position : Outport
  v (m/s) : Outport  Port=2
  wires:
  Constant27/1 -> Divide2/2
  Subtract8/1 -> Scope3/4, Gain18/1  "F_drive (N)"
  Divide2/1 -> Subtract8/1, Scope3/1  "F_avl (N)"
  Integrator5/1 -> Display/1, Index for vehicle position/1, Scope5/1, Operating Cycle/1  "d (m)"
  T_w (Nm)/1 -> Divide2/1
  Gain11/1 -> Subtract8/2, Scope3/2  "F_brake (N)"
  Integrator2/1 -> Saturation1/1  "v (m/s)"
  v_init (m/s)/1 -> Integrator5/2
  Operating Cycle/1 -> Only positive2/1
  Gain18/1 -> Saturation/1  "a (m/s^2)"
  Bpos (0-1)/1 -> Gain4/1
  Gain4/1 -> Gain11/1
  F_res (N)/1 -> Subtract8/3, Scope3/3
  Saturation/1 -> Integrator2/1, To Workspace3/1
  Only positive2/1 -> Scope/1, To Workspace/1  "Vel_target (m/s)"
  Saturation1/1 -> Scope/2, v (m/s)/1, Integrator5/1

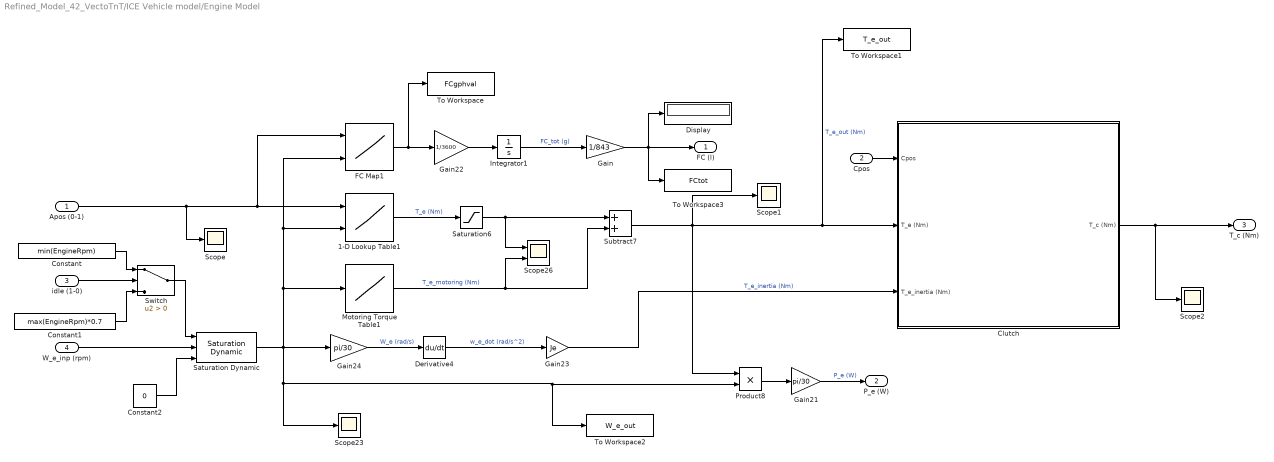
== system Refined_Model_42_VectoTnT/ICE Vehicle model/Engine Model ==
  Apos (0-1) : Inport
  Cpos : Inport  Port=2
  idle (1-0) : Inport  Port=3
  W_e_inp (rpm) : Inport  Port=4
  1-D Lookup Table1 : Lookup_n-D  BreakpointsForDimension1=ThrotPos  BreakpointsForDimension2=RpmBrkPnt  Table=ThrotTableVal  InternalRulePriority=Speed  RndMeth=Simplest  InputSameDT=on
      settings: InputPortMap=u0,u1
  Clutch : Subsystem
  Constant : Constant  Value=min(EngineRpm)
  Constant1 : Constant  Value=max(EngineRpm)*0.7
  Constant2 : Constant  Value=0
  Derivative4 : Derivative
  Display : Display
  FC Map1 : Lookup_n-D  BreakpointsForDimension1=ThrotPos  BreakpointsForDimension2=RpmBrkPnt  Table=FCTableVal  InternalRulePriority=Speed  RndMeth=Simplest  InputSameDT=on
      settings: InputPortMap=u0,u1
  Gain : Gain  Gain=1/843
  Gain21 : Gain  Gain=pi/30
  Gain22 : Gain  Gain=1/3600
  Gain23 : Gain  Gain=Je
  Gain24 : Gain  Gain=pi/30
  Integrator1 : Integrator
  Motoring Torque Table1 : Lookup_n-D  NumberOfTableDimensions=1  BreakpointsForDimension1=EngineRpm  BreakpointsForDimension2=G1Inprpm  Table=MotoringTor  InterpMethod=Linear Lagrange  InternalRulePriority=Speed  RndMeth=Simplest  InputSameDT=on
  Product8 : Product
  Saturation Dynamic : simulink/Discontinuities/Saturation Dynamic  OutMin=[]  OutMax=[]  OutDataTypeStr=Inherit: Same as second input  OutDataType=fixdt(1, 16)  OutScaling=2^-10  DoSatur=off
  Saturation6 : Saturate  UpperLimit=max(ThrotTableVal, [], 'all')  LowerLimit=0
  Scope{,1..2,23} (4 alike) : Scope
  Scope26 : Scope  NumInputPorts=2
  Subtract7 : Sum
  Switch : Switch  Criteria=u2 > Threshold
  To Workspace : ToWorkspace  VariableName=FCgphval  SaveFormat=Timeseries  SampleTime=-1
  To Workspace1 : ToWorkspace  VariableName=T_e_out  SaveFormat=Timeseries  SampleTime=-1
  To Workspace2 : ToWorkspace  VariableName=W_e_out  SaveFormat=Timeseries  SampleTime=-1
  To Workspace3 : ToWorkspace  VariableName=FCtot  SaveFormat=Timeseries  SampleTime=-1
  FC (l) : Outport
  P_e (W) : Outport  Port=2
  T_c (Nm) : Outport  Port=3
  wires:
  Motoring Torque Table1/1 -> Subtract7/2, Scope26/2  "T_e_motoring (Nm)"
  Integrator1/1 -> Gain/1  "FC_tot (g)"
  Derivative4/1 -> Gain23/1  "w_e_dot (rad/s^2)"
  Saturation Dynamic/1 -> Gain24/1, To Workspace2/1, Product8/2, Scope23/1, Motoring Torque Table1/1, 1-D Lookup Table1/2, FC Map1/2
  Product8/1 -> Gain21/1
  Apos (0-1)/1 -> 1-D Lookup Table1/1, FC Map1/1, Scope/1
  1-D Lookup Table1/1 -> Saturation6/1  "T_e (Nm)"
  Gain24/1 -> Derivative4/1  "W_e (rad/s)"
  Gain23/1 -> Clutch/3(T_e_inertia (Nm))  "T_e_inertia (Nm)"
  Gain21/1 -> P_e (W)/1  "P_e (W)"
  Gain22/1 -> Integrator1/1
  Subtract7/1 -> To Workspace1/1, Clutch/2(T_e (Nm)), Scope1/1, Product8/1  "T_e_out (Nm)"
  FC Map1/1 -> To Workspace/1, Gain22/1
  Saturation6/1 -> Scope26/1, Subtract7/1
  Clutch/1(T_c (Nm)) -> Scope2/1, T_c (Nm)/1
  Cpos/1 -> Clutch/1(Cpos)
  Gain/1 -> To Workspace3/1, Display/1, FC (l)/1
  idle (1-0)/1 -> Switch/2
  Constant/1 -> Switch/1
  W_e_inp (rpm)/1 -> Saturation Dynamic/2
  Constant1/1 -> Switch/3
  Switch/1 -> Saturation Dynamic/1
  Constant2/1 -> Saturation Dynamic/3

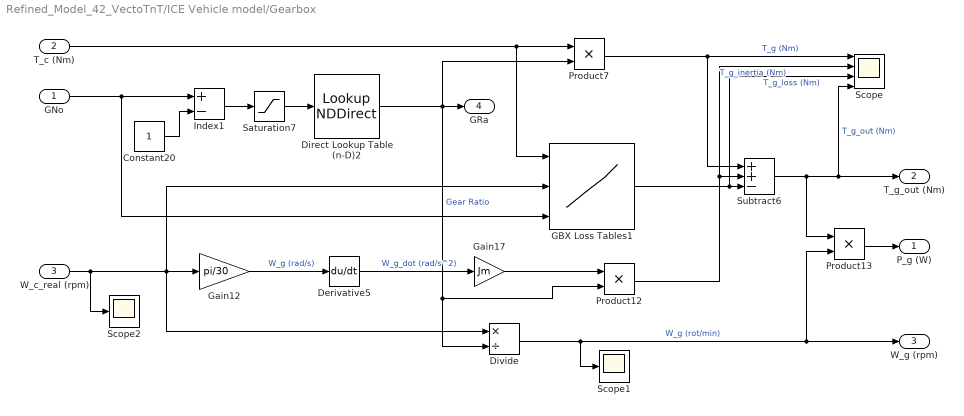
== system Refined_Model_42_VectoTnT/ICE Vehicle model/Gearbox ==
  GNo : Inport
  T_c (Nm) : Inport  Port=2
  W_c_real (rpm) : Inport  Port=3
  Constant20 : Constant
  Derivative5 : Derivative
  Direct Lookup Table (n-D)2 : LookupNDDirect  NumberOfTableDimensions=1  Table=GRa
  Divide : Product  Inputs=*/
  GBX Loss Tables1 : Lookup_n-D  NumberOfTableDimensions=3  BreakpointsForDimension1=GInpTor  BreakpointsForDimension2=GInprpm  BreakpointsForDimension3=GNo  Table=GTorLoss  InterpMethod=Linear Lagrange  InternalRulePriority=Speed  RndMeth=Simplest  InputSameDT=on
      settings: InputPortMap=u0,u1,u2
  Gain12 : Gain  Gain=pi/30
  Gain17 : Gain  Gain=Jm
  Index1 : Sum  Inputs=+-
  Product12 : Product
  Product13 : Product
  Product7 : Product
  Saturation7 : Saturate  UpperLimit=inf  LowerLimit=0
  Scope : Scope  NumInputPorts=4
  Scope1 : Scope
  Scope2 : Scope
  Subtract6 : Sum  Inputs=++-
  P_g (W) : Outport
  T_g_out (Nm) : Outport  Port=2
  W_g (rpm) : Outport  Port=3
  GRa : Outport  Port=4
  wires:
  Product12/1 -> Scope/2, Subtract6/2  "T_g_inertia (Nm)"
  GNo/1 -> Index1/1, GBX Loss Tables1/3
  Gain17/1 -> Product12/1
  T_c (Nm)/1 -> GBX Loss Tables1/1, Product7/1
  Product7/1 -> Subtract6/1, Scope/1  "T_g (Nm)"
  Divide/1 -> Scope1/1, W_g (rpm)/1, Product13/2  "W_g (rot/min)"
  Subtract6/1 -> Scope/4, T_g_out (Nm)/1, Product13/1  "T_g_out (Nm)"
  Derivative5/1 -> Gain17/1  "W_g_dot (rad/s^2)"
  Direct Lookup Table (n-D)2/1 -> GRa/1, Product7/2, Product12/2, Divide/2  "Gear Ratio"
  Saturation7/1 -> Direct Lookup Table (n-D)2/1
  Gain12/1 -> Derivative5/1  "W_g (rad/s)"
  Constant20/1 -> Index1/2
  GBX Loss Tables1/1 -> Scope/3, Subtract6/3  "T_g_loss (Nm)"
  Index1/1 -> Saturation7/1
  Product13/1 -> P_g (W)/1
  W_c_real (rpm)/1 -> Scope2/1, Gain12/1, Divide/1, GBX Loss Tables1/2

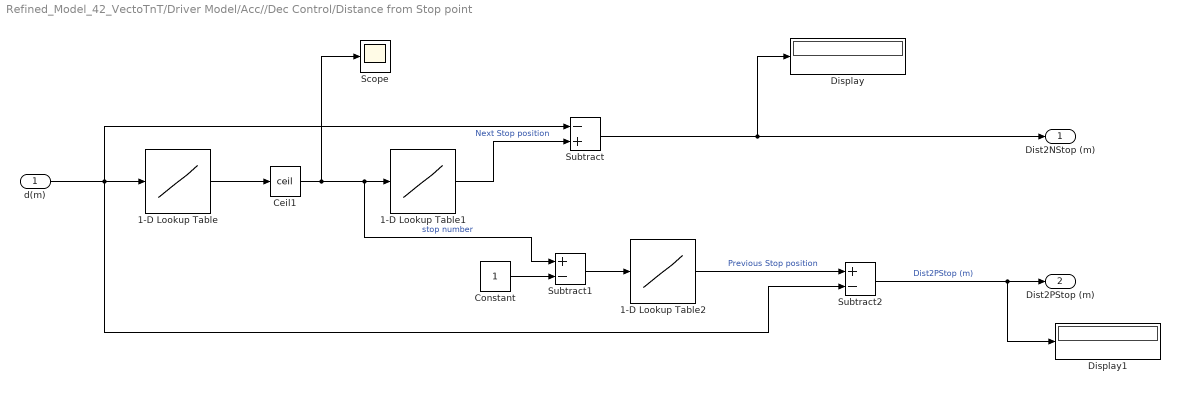
== system Refined_Model_42_VectoTnT/Driver Model/Acc//Dec Control/Distance from Stop point ==
  d(m) : Inport
  1-D Lookup Table : Lookup_n-D  NumberOfTableDimensions=1  BreakpointsForDimension1=Stoptimes(:,1)  Table=1:length(Stoptimes)  InternalRulePriority=Speed  RndMeth=Simplest  InputSameDT=on
  1-D Lookup Table1 : Lookup_n-D  NumberOfTableDimensions=1  BreakpointsForDimension1=1:length(Stoptimes)  Table=Stoptimes(:,1)  InternalRulePriority=Speed  RndMeth=Simplest  InputSameDT=on
  1-D Lookup Table2 : Lookup_n-D  NumberOfTableDimensions=1  BreakpointsForDimension1=1:length(Stoptimes)  Table=Stoptimes(:,1)  InternalRulePriority=Speed  RndMeth=Simplest  InputSameDT=on
  Ceil1 : Rounding  Operator=ceil
  Constant : Constant
  Display : Display
  Display1 : Display
  Scope : Scope
  Subtract : Sum  Inputs=-+
  Subtract1 : Sum  Inputs=+-
  Subtract2 : Sum  Inputs=+-
  Dist2NStop (m) : Outport
  Dist2PStop (m) : Outport  Port=2
  wires:
  1-D Lookup Table2/1 -> Subtract2/1  "Previous Stop position"
  Ceil1/1 -> Scope/1, Subtract1/1, 1-D Lookup Table1/1  "stop number"
  d(m)/1 -> Subtract2/2, Subtract/1, 1-D Lookup Table/1
  Constant/1 -> Subtract1/2
  Subtract1/1 -> 1-D Lookup Table2/1
  1-D Lookup Table/1 -> Ceil1/1
  1-D Lookup Table1/1 -> Subtract/2  "Next Stop position"
  Subtract2/1 -> Display1/1, Dist2PStop (m)/1  "Dist2PStop (m)"
  Subtract/1 -> Display/1, Dist2NStop (m)/1

== system Refined_Model_42_VectoTnT/Driver Model/Acc//Dec Control/Gradient gear limiter ==
  In1 : Inport
  Constant5 : Constant
  Constant6 : Constant  Value=0
  If : If  IfExpression=u1 > 4.5
  If Action Subsystem2 : Subsystem  TreatAsAtomicUnit=on
  If Action Subsystem6 : Subsystem  TreatAsAtomicUnit=on
  Merge : Merge
  Scope : Scope
  Slope (%)1 : Lookup_n-D  NumberOfTableDimensions=1  BreakpointsForDimension1=Dist  Table=IntpSlope  InternalRulePriority=Speed  RndMeth=Simplest  InputSameDT=on
  Out1 : Outport
  wires:
  Constant5/1 -> If Action Subsystem2/1(In1)
  Merge/1 -> Out1/1
  Constant6/1 -> If Action Subsystem6/1(In1)
  If/2 -> If Action Subsystem6/Action
  If Action Subsystem2/1(Out1) -> Merge/1
  Slope (%)1/1 -> Scope/1, If/1
  If/1 -> If Action Subsystem2/Action
  In1/1 -> Slope (%)1/1
  If Action Subsystem6/1(Out1) -> Merge/2

== system Refined_Model_42_VectoTnT/Driver Model/Acc//Dec Control/Stop duration1 ==
  d (m) : Inport
  1-D Lookup Table : Lookup_n-D  NumberOfTableDimensions=1  BreakpointsForDimension1=Stoptimes(:,1)  Table=1:length(Stoptimes)  InternalRulePriority=Speed  RndMeth=Simplest  InputSameDT=on
  Ceil : Rounding  Operator=ceil
  Constant : Constant  Value=10
  Constant2 : Constant
  Direct Lookup Table (n-D) : LookupNDDirect  NumberOfTableDimensions=1  Table=Stoptimes(:,2)
  Scope : Scope
  Scope1 : Scope  NumInputPorts=2
  Scope2 : Scope
  Subtract : Sum  Inputs=+-
  Subtract1 : Sum  Inputs=+-
  Stop_t (s) : Outport
  wires:
  1-D Lookup Table/1 -> Scope1/1, Ceil/1
  d (m)/1 -> Subtract/1, Scope2/1
  Subtract1/1 -> Direct Lookup Table (n-D)/1
  Direct Lookup Table (n-D)/1 -> Stop_t (s)/1, Scope/1  "Stop time (s)"
  Ceil/1 -> Scope1/2, Subtract1/1
  Constant2/1 -> Subtract1/2
  Subtract/1 -> 1-D Lookup Table/1
  Constant/1 -> Subtract/2

== system Refined_Model_42_VectoTnT/Driver Model/Acc//Dec Control/Stopping distance calc ==
  v (m/s) : Inport
  Add : Sum
  Constant2 : Constant  Value=0
  Constant4 : Constant  Value=MaxDec
  Divide : Product  Inputs=*/
  Gain : Gain  Gain=2
  Gain1 : Gain  Gain=0.01
  Gain2 : Gain  Gain=-1
  Magnitude Squared : Math  Operator=square  SaturateOnIntegerOverflow=on
  Magnitude Squared1 : Math  Operator=square  SaturateOnIntegerOverflow=on
  Scope : Scope
  Subtract1 : Sum  Inputs=+-
  Dist2Dec (m) : Outport
  wires:
  Divide/1 -> Add/2, Gain1/1  "Dist2Dec (m)"
  Subtract1/1 -> Divide/1
  Magnitude Squared1/1 -> Subtract1/2
  Constant4/1 -> Gain2/1  "deceleration in m/s^2"
  Magnitude Squared/1 -> Subtract1/1
  Gain/1 -> Divide/2
  Gain2/1 -> Gain/1
  Constant2/1 -> Magnitude Squared/1
  v (m/s)/1 -> Magnitude Squared1/1
  Gain1/1 -> Add/1
  Add/1 -> Scope/1, Dist2Dec (m)/1

== system Refined_Model_42_VectoTnT/Driver Model/Acc//Dec Control/Trip complete ==
  d (m) : Inport
  Abs : Abs
  Constant1 : Constant  Value=NoSteps
  Constant2 : Constant
  Delay : Delay  DelayLength=1
  Derivative : Derivative
  If : If  NumInputs=2  IfExpression=u1 <= 200 & u2 ==0  ShowElse=off
  If Action Subsystem : Subsystem  TreatAsAtomicUnit=on
  Max : MinMax  Function=max
  Stop Simulation : Stop
  Subtract : Sum  Inputs=+-
  wires:
  Constant1/1 -> Subtract/2
  Constant2/1 -> If Action Subsystem/1(In1)
  If/1 -> If Action Subsystem/Action
  If Action Subsystem/1(Out1) -> Delay/1
  d (m)/1 -> Max/1, Derivative/1
  Delay/1 -> Stop Simulation/1
  Derivative/1 -> If/2  "v (m/s)"
  Max/1 -> Subtract/1
  Subtract/1 -> Abs/1
  Abs/1 -> If/1

== system Refined_Model_42_VectoTnT/Driver Model/Acc//Dec Control/Upcoming speed ==
  d (m) : Inport
  Add3 : Sum
  Ceil : Rounding  Operator=ceil
  Constant : Constant
  Saturation1 : Saturate  UpperLimit=inf  LowerLimit=0
  Saturation2 : Saturate  UpperLimit=inf  LowerLimit=0
  Scope : Scope
  Segment number : Lookup_n-D  NumberOfTableDimensions=1  BreakpointsForDimension1=CovDist  BreakpointsForDimension2=G1Inprpm  Table=SegNo  InterpMethod=Linear Lagrange  InternalRulePriority=Speed  RndMeth=Simplest  InputSameDT=on
  upcoming speed (m/s) : Lookup_n-D  NumberOfTableDimensions=1  BreakpointsForDimension1=SegNo  BreakpointsForDimension2=G1Inprpm  Table=SegSPLatinmps  InterpMethod=Linear Lagrange  InternalRulePriority=Speed  RndMeth=Simplest  InputSameDT=on
  UpSp (m/s) : Outport
  wires:
  upcoming speed (m/s)/1 -> Saturation1/1
  Ceil/1 -> Add3/1
  Constant/1 -> Add3/2
  Add3/1 -> upcoming speed (m/s)/1
  d (m)/1 -> Segment number/1
  Saturation1/1 -> Scope/1, UpSp (m/s)/1
  Segment number/1 -> Saturation2/1
  Saturation2/1 -> Ceil/1

== system Refined_Model_42_VectoTnT/Driver Model/Driver Throttle Mapping ICE/Idling// Apos = 0 ==
  Apos(m/s^2) : Inport
  Constant : Constant
  Constant2 : Constant  Value=0
  Idling : If  IfExpression=u1 == 0
  If Action Subsystem : Subsystem  TreatAsAtomicUnit=on
  If Action Subsystem1 : Subsystem  TreatAsAtomicUnit=on
  Merge : Merge
  Azero : Outport
  wires:
  Constant2/1 -> If Action Subsystem1/1(In1)
  Idling/1 -> If Action Subsystem/Action
  Merge/1 -> Azero/1
  If Action Subsystem1/1(Out1) -> Merge/1
  Constant/1 -> If Action Subsystem/1(In1)
  Apos(m/s^2)/1 -> Idling/1
  Idling/2 -> If Action Subsystem1/Action
  If Action Subsystem/1(Out1) -> Merge/2

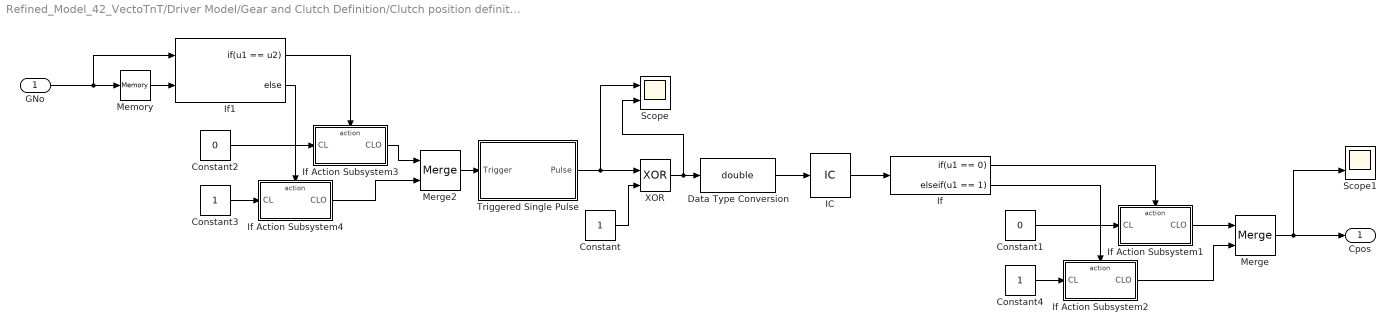
== system Refined_Model_42_VectoTnT/Driver Model/Gear and Clutch Definition/Clutch position definition ==
  GNo : Inport
  Constant : Constant
  Constant1 : Constant  Value=0
  Constant2 : Constant  Value=0
  Constant3 : Constant
  Constant4 : Constant
  Data Type Conversion : DataTypeConversion  OutDataTypeStr=double
  IC : InitialCondition  Value=0
  If : If  IfExpression=u1 == 0  ElseIfExpressions=u1 == 1  ShowElse=off
  If Action Subsystem1 : Subsystem  TreatAsAtomicUnit=on
  If Action Subsystem2 : Subsystem  TreatAsAtomicUnit=on
  If Action Subsystem3 : Subsystem  TreatAsAtomicUnit=on
  If Action Subsystem4 : Subsystem  TreatAsAtomicUnit=on
  If1 : If  NumInputs=2  IfExpression=u1 == u2
  Memory : Memory
  Merge : Merge
  Merge2 : Merge
  Scope : Scope  NumInputPorts=2
  Scope1 : Scope  NumInputPorts=2
  Triggered Single Pulse : Subsystem  TreatAsAtomicUnit=on  mask(single pulse generation){p_wid=2}
      mask prompts: p_wid "pulse width (number of samples)"
      mask help: This block generate a single pulse whenever a trigger happen. The pulse width must specified as a number of samples. for example if your sampling time is 0.1s and you want 3s pulse , then you should enter 30 as a pulse width.
      mask Display:
      | plot([0],[0])
      | plot([11],[0])
      | plot([5],[0.5])
      | plot([4 5 5 6 6 7],[0 0 0.25 0.25 0 0])
      | plot([5],[-0.3])
      | 
      | port_label('output', 1, 'Pulse')
      | port_label('input', 1, 'Trigger')
  XOR : Logic  Operator=XOR  IconShape=distinctive  AllPortsSameDT=off  OutDataTypeStr=boolean
  Cpos : Outport
  wires:
  If1/1 -> If Action Subsystem3/Action
  If Action Subsystem3/1(CLO) -> Merge2/1
  Memory/1 -> If1/2
  Constant2/1 -> If Action Subsystem3/1(CL)
  Constant3/1 -> If Action Subsystem4/1(CL)
  GNo/1 -> Memory/1, If1/1
  If1/2 -> If Action Subsystem4/Action
  If Action Subsystem4/1(CLO) -> Merge2/2
  Merge2/1 -> Triggered Single Pulse/1(Trigger)
  Triggered Single Pulse/1(Pulse) -> Scope/1, XOR/1
  Constant/1 -> XOR/2
  XOR/1 -> Scope/2, Data Type Conversion/1
  Data Type Conversion/1 -> IC/1
  IC/1 -> If/1
  Constant4/1 -> If Action Subsystem2/1(CL)
  Constant1/1 -> If Action Subsystem1/1(CL)
  If Action Subsystem2/1(CLO) -> Merge/2
  If/2 -> If Action Subsystem2/Action
  If/1 -> If Action Subsystem1/Action
  If Action Subsystem1/1(CLO) -> Merge/1
  Merge/1 -> Scope1/2, Cpos/1

== system Refined_Model_42_VectoTnT/Driver Model/Gear and Clutch Definition/Gradient gear limiter ==
  In1 : Inport
  Constant5 : Constant
  Constant6 : Constant  Value=0
  If : If  IfExpression=u1 > 4.5
  If Action Subsystem2 : Subsystem  TreatAsAtomicUnit=on
  If Action Subsystem6 : Subsystem  TreatAsAtomicUnit=on
  Integrator : Integrator
  Merge : Merge
  Slope (%) : Lookup_n-D  NumberOfTableDimensions=1  BreakpointsForDimension1=Dist  Table=IntpSlope  InternalRulePriority=Speed  RndMeth=Simplest  InputSameDT=on
  Out1 : Outport
  wires:
  Constant6/1 -> If Action Subsystem6/1(In1)
  If/2 -> If Action Subsystem6/Action
  Constant5/1 -> If Action Subsystem2/1(In1)
  Slope (%)/1 -> If/1
  Merge/1 -> Out1/1
  Integrator/1 -> Slope (%)/1
  If Action Subsystem6/1(Out1) -> Merge/2
  If Action Subsystem2/1(Out1) -> Merge/1
  If/1 -> If Action Subsystem2/Action
  In1/1 -> Integrator/1

== system Refined_Model_42_VectoTnT/Driver Model/Gear and Clutch Definition/If Action Subsystem ==
  In1 : Inport
  Action Port : ActionPort  ActionPortLabel=elseif( u1 == 0)
  Out1 : Outport
  wires:
  In1/1 -> Out1/1

== system Refined_Model_42_VectoTnT/Driver Model/Gear and Clutch Definition/If Action Subsystem1 ==
  Selected Gear /dt : Inport
  Action Port : ActionPort  ActionPortLabel=elseif(u2 <= -0.2)
  Constant : Constant
  Subtract : Sum  Inputs=+-
  Decreased gear : Outport
  wires:
  Constant/1 -> Subtract/2
  Subtract/1 -> Decreased gear/1
  Selected Gear /dt/1 -> Subtract/1

== system Refined_Model_42_VectoTnT/Driver Model/Gear and Clutch Definition/If Action Subsystem3 ==
  Selected Gear /dt : Inport
  Action Port : ActionPort  ActionPortLabel=if(u1 >= u3)
  Add : Sum
  Constant : Constant
  Increased gear : Outport
  wires:
  Selected Gear /dt/1 -> Add/1
  Add/1 -> Increased gear/1
  Constant/1 -> Add/2

== system Refined_Model_42_VectoTnT/Driver Model/Gear and Clutch Definition/If Action Subsystem4 ==
  Selected Gear /dt : Inport
  Action Port : ActionPort  ActionPortLabel=elseif(u4 >= u5 )
  Constant : Constant
  Subtract : Sum  Inputs=+-
  Decreased gear : Outport
  wires:
  Constant/1 -> Subtract/2
  Subtract/1 -> Decreased gear/1
  Selected Gear /dt/1 -> Subtract/1

== system Refined_Model_42_VectoTnT/Driver Model/Gear and Clutch Definition/If Action Subsystem5 ==
  Selected Gear Ratio /dt : Inport
  Action Port : ActionPort  ActionPortLabel=else
  Out1 : Outport
  wires:
  Selected Gear Ratio /dt/1 -> Out1/1

== system Refined_Model_42_VectoTnT/ICE Vehicle model/Engine Model/Clutch ==
  Cpos : Inport
  T_e (Nm) : Inport  Port=2
  T_e_inertia (Nm) : Inport  Port=3
  Add : Sum
  Clutch value1 : Product
  Gain20 : Gain  Gain=etaClutch
  Saturation2 : Saturate  UpperLimit=inf  LowerLimit=0
  Scope : Scope
  Scope1 : Scope  NumInputPorts=2
  T_c (Nm) : Outport
  wires:
  Cpos/1 -> Clutch value1/1
  Clutch value1/1 -> Gain20/1
  Gain20/1 -> Saturation2/1  "T_c (Nm)"
  T_e_inertia (Nm)/1 -> Add/2, Scope1/2
  T_e (Nm)/1 -> Add/1
  Saturation2/1 -> Scope/1, T_c (Nm)/1
  Add/1 -> Scope1/1, Clutch value1/2

== system Refined_Model_42_VectoTnT/Driver Model/Acc//Dec Control/Gradient gear limiter/If Action Subsystem2 ==
  In1 : Inport
  Action Port : ActionPort  ActionPortLabel=if(u1 > 4.5)
  Out1 : Outport
  wires:
  In1/1 -> Out1/1

== system Refined_Model_42_VectoTnT/Driver Model/Acc//Dec Control/Gradient gear limiter/If Action Subsystem6 ==
  In1 : Inport
  Action Port : ActionPort  ActionPortLabel=else
  Out1 : Outport
  wires:
  In1/1 -> Out1/1

== system Refined_Model_42_VectoTnT/Driver Model/Acc//Dec Control/Trip complete/If Action Subsystem ==
  In1 : Inport
  Action Port : ActionPort  ActionPortLabel=if(u1 <= 200 & u2 ==0)
  Out1 : Outport
  wires:
  In1/1 -> Out1/1

== system Refined_Model_42_VectoTnT/Driver Model/Driver Throttle Mapping ICE/Idling// Apos = 0/If Action Subsystem ==
  In1 : Inport
  Action Port : ActionPort  ActionPortLabel=if(u1 == 0)
  Out1 : Outport
  wires:
  In1/1 -> Out1/1

== system Refined_Model_42_VectoTnT/Driver Model/Driver Throttle Mapping ICE/Idling// Apos = 0/If Action Subsystem1 ==
  In1 : Inport
  Action Port : ActionPort  ActionPortLabel=else
  Out1 : Outport
  wires:
  In1/1 -> Out1/1

== system Refined_Model_42_VectoTnT/Driver Model/Gear and Clutch Definition/Clutch position definition/If Action Subsystem1 ==
  CL : Inport
  Action Port : ActionPort  ActionPortLabel=if(u1 == 0)
  CLO : Outport
  wires:
  CL/1 -> CLO/1

== system Refined_Model_42_VectoTnT/Driver Model/Gear and Clutch Definition/Clutch position definition/If Action Subsystem2 ==
  CL : Inport
  Action Port : ActionPort  ActionPortLabel=elseif(u1 == 1)
  CLO : Outport
  wires:
  CL/1 -> CLO/1

== system Refined_Model_42_VectoTnT/Driver Model/Gear and Clutch Definition/Clutch position definition/If Action Subsystem3 ==
  CL : Inport
  Action Port : ActionPort  ActionPortLabel=if(u1 == u2)
  CLO : Outport
  wires:
  CL/1 -> CLO/1

== system Refined_Model_42_VectoTnT/Driver Model/Gear and Clutch Definition/Clutch position definition/If Action Subsystem4 ==
  CL : Inport
  Action Port : ActionPort  ActionPortLabel=else
  CLO : Outport
  wires:
  CL/1 -> CLO/1

== system Refined_Model_42_VectoTnT/Driver Model/Gear and Clutch Definition/Clutch position definition/Triggered Single Pulse ==
  Trigger : Inport
  +ve edge detect : Subsystem
  Add : Sum
  Add1 : Sum
  Compare To Constant : simulink/Logic and Bit Operations/Compare To Constant  relop=>  const=p_wid-1  OutDataTypeStr=boolean
  Constant2 : Constant
  Logical Operator : Logic  Operator=NOT  AllPortsSameDT=off  OutDataTypeStr=boolean
  Product : Product  RndMeth=Zero
  Product1 : Product  RndMeth=Zero
  Product3 : Product  RndMeth=Zero
  Saturation : Saturate  UpperLimit=1  LowerLimit=0
  Unit Delay : UnitDelay  SampleTime=-1  HasFrameUpgradeWarning=on
  Unit Delay1 : UnitDelay  SampleTime=-1  HasFrameUpgradeWarning=on
  Pulse : Outport
  wires:
  Compare To Constant/1 -> Logical Operator/1
  Constant2/1 -> Product/1
  Product/1 -> Add/1
  Unit Delay/1 -> Add/2, Compare To Constant/1
  Trigger/1 -> +ve edge detect/1(signal)
  +ve edge detect/1(out) -> Add1/2
  Add/1 -> Product1/2
  Product1/1 -> Unit Delay/1
  Add1/1 -> Unit Delay1/1
  Unit Delay1/1 -> Saturation/1
  Saturation/1 -> Product3/1
  Product3/1 -> Add1/1, Product/2, Product1/1, Pulse/1
  Logical Operator/1 -> Product3/2

== system Refined_Model_42_VectoTnT/Driver Model/Gear and Clutch Definition/Gradient gear limiter/If Action Subsystem2 ==
  In1 : Inport
  Action Port : ActionPort  ActionPortLabel=if(u1 > 4.5)
  Out1 : Outport
  wires:
  In1/1 -> Out1/1

== system Refined_Model_42_VectoTnT/Driver Model/Gear and Clutch Definition/Gradient gear limiter/If Action Subsystem6 ==
  In1 : Inport
  Action Port : ActionPort  ActionPortLabel=else
  Out1 : Outport
  wires:
  In1/1 -> Out1/1

== system Refined_Model_42_VectoTnT/Driver Model/Gear and Clutch Definition/Clutch position definition/Triggered Single Pulse/+ve edge detect ==
  note: Edge
  signal : Inport
  Delay Input1 : UnitDelay  Description=Store in Global RAM  DisableCoverage=on  SampleTime=-1  HasFrameUpgradeWarning=on
  FixPt Relational Operator : RelationalOperator  Operator=>  OutDataTypeStr=fixdt(0, 8)  ZeroCross=off  RndMeth=Nearest
  Positive : simulink/Logic and Bit Operations/Compare To Zero  relop=>  OutDataTypeStr=uint8  ZeroCross=off
  out : Outport
  wires:
  Delay Input1/1 -> FixPt Relational Operator/2  "U(k-1)"
  Positive/1 -> Delay Input1/1, FixPt Relational Operator/1  "U(k)"
  FixPt Relational Operator/1 -> out/1
  signal/1 -> Positive/1

== stateflow chart Refined_Model_42_VectoTnT/Driver Model/Acc//Dec Control/Driving State ==
  state Driving
    idle = 0;
    Bor = 0;
    Aor = 1;
    error = x;
  state Stopping
    idle = 0;
    Bor = 1;
    Aor = 0;
    error = x;
  state Calibration_nve
    idle = 1;
    Bor = 1;
    Aor = 0;
    x = Dist2PStop;
  state Idling
    idle = 1;
    Bor = 1;
    Aor = 0;
    error = x;
  state Calibration_pve
    idle = 1;
    Bor = 1;
    Aor = 0;
    x = Dist2NStop;
  (default) -> Driving : {x = 0;}
  Driving -> Stopping : [Dist2NStop <= Dist2Dec && UpSp <= v]
  Stopping -> Calibration_nve [order 2] : [v == 0 && d > 0 && Dist2PStop <= 25 && Dist2Dec <= 0]{Bor = 1;}
  Idling -> Driving : after(Stoptime/3.7,sec) [a == 0]{Aor == 1}
  Stopping -> Calibration_pve [order 1] : [v == 0 && d > 0 && Dist2NStop <= 25 && Dist2Dec == 0]{Bor = 1;}
  Calibration_pve -> Idling : [v == 0]{idle = 1;Bor = 1;x = x + Dist2NStop}
  Calibration_nve -> Idling : [v == 0 ]{idle = 1;Bor = 1;x = x - Dist2PStop}
  data: v input; a input; d input; idle output =0; Bor output; Stoptime input; Dist2NStop input; Dist2Dec input; UpSp input; Aor output; Dist2PStop input; x output double =0; error local
